simulink model "chap9_4sim"  (Simulink 5.0)
settings: Solver=ode45  StartTime=0.0  StopTime=10  FixedStep=0.00000010  RelTol=1e-3
settings Model: LastModifiedBy=Administrator  ExtModeTrigMode=oneshot  ExtModeArmWhenConnect=off  LimitDataPoints=off  BooleanDataType=off

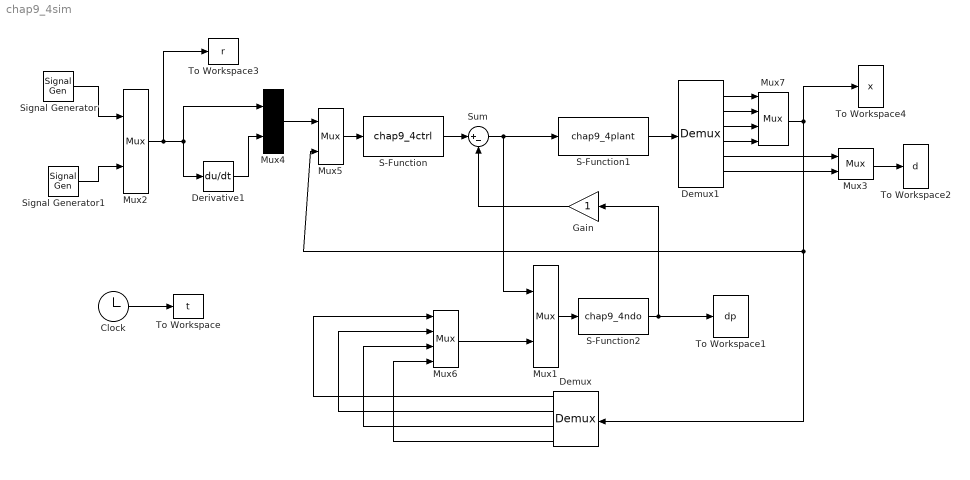
== system chap9_4sim ==
  Clock : Clock
  Demux : Demux  Orientation=left
  Demux1 : Demux  Outputs=6
  Derivative1 : Derivative
  Gain : Gain  Orientation=left  SaturateOnIntegerOverflow=on
  Mux{1..5} (5 alike) : Mux  Inputs=2
  Mux6 : Mux
  Mux7 : Mux
  S-Function : S-Function  FunctionName=chap9_4ctrl
  S-Function1 : S-Function  FunctionName=chap9_4plant
  S-Function2 : S-Function  FunctionName=chap9_4ndo
  Signal Generator : SignalGenerator  Frequency=0.1
  Signal Generator1 : SignalGenerator  Frequency=0.1
  Sum : Sum  Inputs=|+-  SaturateOnIntegerOverflow=on
  To Workspace : ToWorkspace  VariableName=t  SampleTime=-1  SaveFormat=Array
  To Workspace1 : ToWorkspace  VariableName=dp  SampleTime=-1  SaveFormat=Array
  To Workspace2 : ToWorkspace  VariableName=d  SampleTime=-1  SaveFormat=Array
  To Workspace3 : ToWorkspace  VariableName=r  SampleTime=-1  SaveFormat=Array
  To Workspace4 : ToWorkspace  VariableName=x  SampleTime=-1  SaveFormat=Array
  wires:
  Signal Generator/1 -> Mux2/1
  Signal Generator1/1 -> Mux2/2
  Clock/1 -> To Workspace/1
  Mux1/1 -> S-Function2/1
  S-Function2/1 -> To Workspace1/1, Gain/1
  Mux2/1 -> Derivative1/1, Mux4/1, To Workspace3/1
  Mux5/1 -> S-Function/1
  Mux4/1 -> Mux5/1
  Derivative1/1 -> Mux4/2
  Mux6/1 -> Mux1/2
  Demux/2 -> Mux6/2
  Demux/1 -> Mux6/1
  Demux/3 -> Mux6/3
  Demux/4 -> Mux6/4
  S-Function1/1 -> Demux1/1
  Demux1/1 -> Mux7/1
  Demux1/2 -> Mux7/2
  Demux1/3 -> Mux7/3
  Demux1/4 -> Mux7/4
  Mux7/1 -> Demux/1, Mux5/2, To Workspace4/1
  Demux1/5 -> Mux3/1
  Demux1/6 -> Mux3/2
  Mux3/1 -> To Workspace2/1
  S-Function/1 -> Sum/1
  Sum/1 -> S-Function1/1, Mux1/1
  Gain/1 -> Sum/2
